simulink model "UUV_PID"  (Simulink 8.3)
settings: Solver=ode45  StartTime=0.0  StopTime=10  RelTol=1e-3
values from neighbouring files (symbols this model uses):
  P = [-1.2-1.8j -1.2+1.8j]    [UUV_roll_ctrl.m]
undefined symbols (not defined in the file or in its folder): drawUUV, UUV_roll_ctrl
settings Model: Creator=beard  LastModifiedBy=jhl48
settings OptimizationCC: ExpressionDepthLimit=2147483647  InitFltsAndDblsToZero=on
settings DebuggingCC: FcnCallInpInsideContextMsg=UseLocalSettings

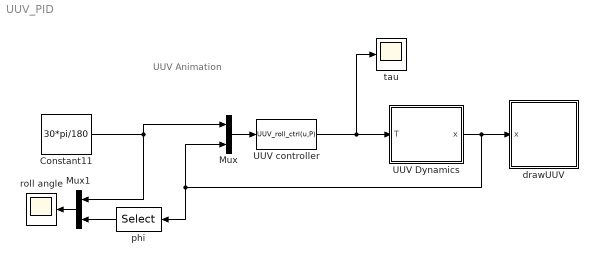
== system UUV_PID ==
  note: UUV Animation
  Constant11 : Constant  Value=30*pi/180
  Mux : Mux  Inputs=2
  Mux1 : Mux  Inputs=2
  UUV Dynamics : Subsystem
  UUV controller : MATLABFcn  MATLABFcn=UUV_roll_ctrl(u,P)  OutputDimensions=1  SampleTime=P.Ts
  drawUUV : Subsystem
      mask init:
      | % drawing parameters
      | MajorAxis = 10;
      | MinorAxis = 6;
      | C_M = [0;-4];
      mask Display: image(imread('tv.jpg'))
  phi : Selector  InputPortWidth=2  Indices=[1]
  roll angle : Scope
      settings: TimeRange=16  YMin=-1.5e-14  YMax=5e-14  SaveName=ScopeData2
  tau : Scope
      settings: TimeRange=40  YMin=-80  YMax=0
  wires:
  UUV controller/1 -> UUV Dynamics/1(T), tau/1
  Mux/1 -> UUV controller/1
  UUV Dynamics/1(x) -> Mux/2, phi/1, drawUUV/1(x)
  Mux1/1 -> roll angle/1
  Constant11/1 -> Mux/1, Mux1/1
  phi/1 -> Mux1/2

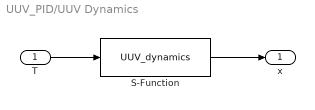
== system UUV_PID/UUV Dynamics ==
  T : Inport
  S-Function : S-Function  FunctionName=UUV_dynamics  Parameters=P  EnableBusSupport=off
  x : Outport
  wires:
  T/1 -> S-Function/1
  S-Function/1 -> x/1

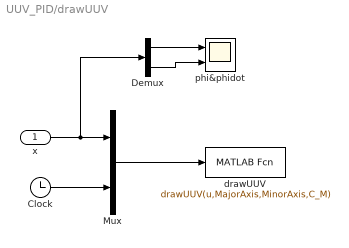
== system UUV_PID/drawUUV ==
  x : Inport
  Clock : Clock
  Demux : Demux  Outputs=2
  Mux : Mux  Inputs=2
  drawUUV : MATLABFcn  MATLABFcn=drawUUV(u,MajorAxis,MinorAxis,C_M)  OutputDimensions=0  SampleTime=0.1
  phi&phidot : Scope  NumInputPorts=2
      settings: TimeRange=40  YMin=0~0  YMax=0.8~0.4
  wires:
  Mux/1 -> drawUUV/1
  x/1 -> Mux/1, Demux/1
  Clock/1 -> Mux/2
  Demux/1 -> phi&phidot/1
  Demux/2 -> phi&phidot/2
